simulink model "tests"  (R2013a)
settings: Solver=ode45  StartTime=0.0  StopTime=1  MaxStep=1e-3  RelTol=1e-3
undefined symbols (not defined in the file or in its folder): Nadc
libraries: simulink x1
settings Model: Creator=mainster  LastModifiedBy=mainster

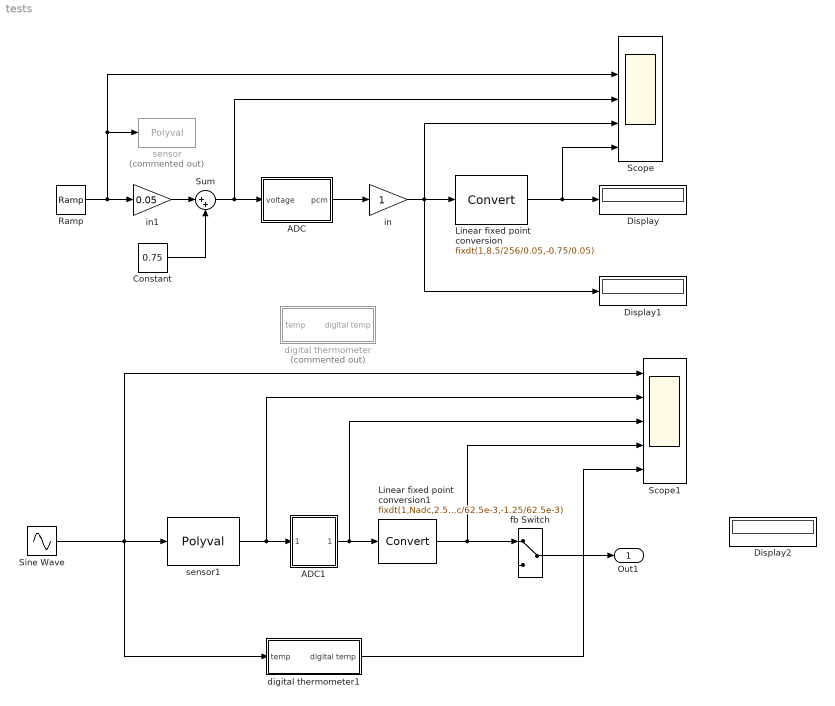
== system tests ==
  ADC : Subsystem
      mask Display: fprintf('ADC\n8-bit\n0-5V');
  ADC1 : Subsystem  mask{bypass=off}
      mask prompts: bypass "bypass adc"
      mask Callback bypass: %Simulink.Block.eval([gcb '/switch']);
      mask Display:
      | %fprintf('ADC\nGain=%s\n=%i',...
      | %    get_param([gcb '/scale'], 'Gain'),...
      | %    eval( get_param([gcb '/scale'], 'Gain') ));
      | if bypass
      |     color('red')
      |     fprintf('bypass\nADC')
      | else
      |     color('black')
      |     fprintf('ADC')
      | end
  Constant : Constant  Value=0.75
  Display : Display
  Display1 : Display
  Display2 : Display
  Linear fixed point conversion : DataTypeConversion  OutDataTypeStr=fixdt(1,8,5/256/0.05,-0.75/0.05)  ConvertRealWorld=Stored Integer (SI)
  Linear fixed point conversion1 : DataTypeConversion  OutDataTypeStr=fixdt(1,Nadc,2.5/2^Nadc/62.5e-3,-1.25/62.5e-3)  ConvertRealWorld=Stored Integer (SI)
  Ramp : simulink/Sources/Ramp  slope=50  start=0  X0=-5
  Scope : Scope  NumInputPorts=5
      settings: ShowLegends=on  TimeRange=1  YMin=-1~-10~0.5~0~-80  YMax=1~50~3~200~40
  Scope1 : Scope  NumInputPorts=5
      settings: ShowLegends=on  TimeRange=0.08057851239669417  YMin=-20~-10~-150~-3~-20  YMax=20~10~150~3~30
  Sine Wave : Sin  Amplitude=15  Frequency=2*pi  SampleTime=0
  Sum : Sum  Inputs=|++
  digital thermometer : Subsystem  Commented=on
  digital thermometer1 : Subsystem
  fb Switch : ManualSwitch
  in : Gain
  in1 : Gain  Gain=0.05
  sensor : Polyval  Commented=on  Coefs="[ 0.05     0.75 ]"
  sensor1 : Polyval  Coefs="[ 1/16    1.25]"
  Out1 : Outport
  wires:
  Linear fixed point conversion/1 -> Scope/5, Display/1
  ADC/1(pcm) -> in/1
  in/1 -> Scope/4, Display1/1, Linear fixed point conversion/1
  Ramp/1 -> Scope/2, sensor/1, in1/1
  Constant/1 -> Sum/2
  Sum/1 -> Scope/3, ADC/1(voltage)
  in1/1 -> Sum/1
  sensor1/1 -> ADC1/1(voltage), Scope1/2
  Sine Wave/1 -> digital thermometer1/1(temp), Scope1/1, sensor1/1
  fb Switch/1 -> Out1/1
  Linear fixed point conversion1/1 -> Scope1/4, fb Switch/1
  ADC1/1(pcm) -> Scope1/3, Linear fixed point conversion1/1
  digital thermometer1/1(digital temp) -> Scope1/5

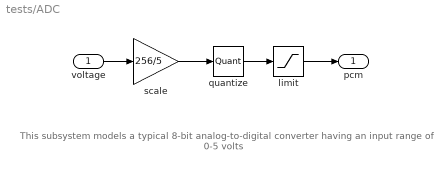
== system tests/ADC ==
  note: This subsystem models a typical
      | 8-bit analog-to-digital converter
      | having an input range of 0-5 volts
  voltage : Inport
  limit : Saturate  UpperLimit=255  LowerLimit=0
  quantize : Quantizer  QuantizationInterval=1
  scale : Gain  Gain=256/5  SaturateOnIntegerOverflow=on  OutDataTypeStr=Inherit: Same as input  ParamDataTypeStr=Inherit: Same as input
  pcm : Outport
  wires:
  limit/1 -> pcm/1
  scale/1 -> quantize/1
  quantize/1 -> limit/1
  voltage/1 -> scale/1

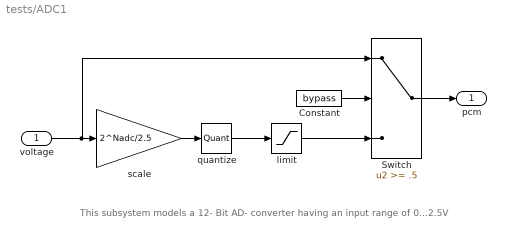
== system tests/ADC1 ==
  note: This subsystem models a 12- Bit AD- converter
      | having an input  range of 0...2.5V
  voltage : Inport
  Constant : Constant  Value=bypass
  Switch : Switch  Threshold=.5
  limit : Saturate  UpperLimit=2^Nadc-1  LowerLimit=0
  quantize : Quantizer
  scale : Gain  Gain=2^Nadc/2.5  SaturateOnIntegerOverflow=on  OutDataTypeStr=Inherit: Same as input  ParamDataTypeStr=Inherit: Same as input
  pcm : Outport
  wires:
  limit/1 -> Switch/3
  scale/1 -> quantize/1
  quantize/1 -> limit/1
  voltage/1 -> Switch/1, scale/1
  Constant/1 -> Switch/2
  Switch/1 -> pcm/1

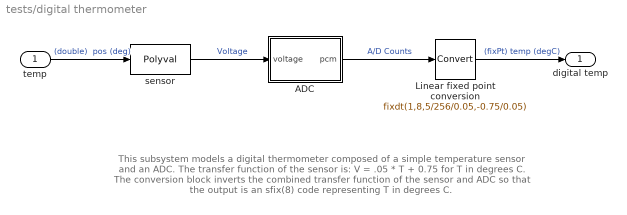
== system tests/digital thermometer ==
  note: This subsystem models a digital thermometer composed of a simple
      | temperature sensor and an ADC.  The transfer function of the sensor is:
      | V = .05 * T + 0.75
      | for T in degrees C.
      |
      | The conversion block inverts the combined transfer function of the sensor
      | and ADC so that the output is an sfix(8) code representing T in degrees C.
  temp : Inport
  ADC : Subsystem
      mask Display: fprintf('ADC\n8-bit\n0-5V');
  Linear fixed point conversion : DataTypeConversion  OutDataTypeStr=fixdt(1,8,5/256/0.05,-0.75/0.05)  ConvertRealWorld=Stored Integer (SI)
  sensor : Polyval  Coefs="[ 2     0 ]"
  digital temp : Outport
  wires:
  sensor/1 -> ADC/1(voltage)  "Voltage"
  ADC/1(pcm) -> Linear fixed point conversion/1  "A/D Counts"
  temp/1 -> sensor/1  "(double)  pos (deg)"
  Linear fixed point conversion/1 -> digital temp/1  "(fixPt) temp (degC)"

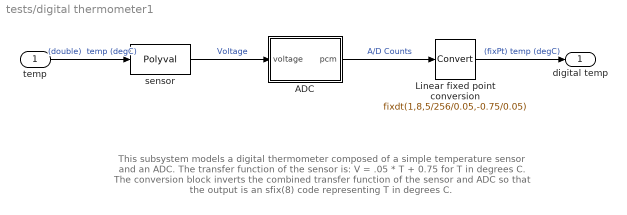
== system tests/digital thermometer1 ==
  note: This subsystem models a digital thermometer composed of a simple
      | temperature sensor and an ADC.  The transfer function of the sensor is:
      | V = .05 * T + 0.75
      | for T in degrees C.
      |
      | The conversion block inverts the combined transfer function of the sensor
      | and ADC so that the output is an sfix(8) code representing T in degrees C.
  temp : Inport
  ADC : Subsystem
      mask Display: fprintf('ADC\n8-bit\n0-5V');
  Linear fixed point conversion : DataTypeConversion  OutDataTypeStr=fixdt(1,8,5/256/0.05,-0.75/0.05)  ConvertRealWorld=Stored Integer (SI)
  sensor : Polyval  Coefs="[ 0.05     0.75 ]"
  digital temp : Outport
  wires:
  sensor/1 -> ADC/1(voltage)  "Voltage"
  ADC/1(pcm) -> Linear fixed point conversion/1  "A/D Counts"
  temp/1 -> sensor/1  "(double)  temp (degC)"
  Linear fixed point conversion/1 -> digital temp/1  "(fixPt) temp (degC)"

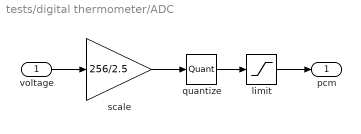
== system tests/digital thermometer/ADC ==
  voltage : Inport
  limit : Saturate  UpperLimit=255  LowerLimit=0
  quantize : Quantizer  QuantizationInterval=1
  scale : Gain  Gain=256/2.5  SaturateOnIntegerOverflow=on  OutDataTypeStr=Inherit: Same as input  ParamDataTypeStr=Inherit: Same as input
  pcm : Outport
  wires:
  limit/1 -> pcm/1
  scale/1 -> quantize/1
  quantize/1 -> limit/1
  voltage/1 -> scale/1

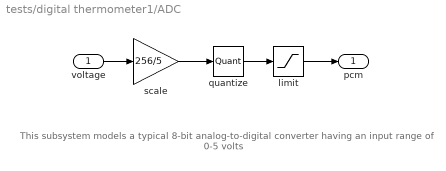
== system tests/digital thermometer1/ADC ==
  note: This subsystem models a typical
      | 8-bit analog-to-digital converter
      | having an input range of 0-5 volts
  voltage : Inport
  limit : Saturate  UpperLimit=255  LowerLimit=0
  quantize : Quantizer  QuantizationInterval=1
  scale : Gain  Gain=256/5  SaturateOnIntegerOverflow=on  OutDataTypeStr=Inherit: Same as input  ParamDataTypeStr=Inherit: Same as input
  pcm : Outport
  wires:
  limit/1 -> pcm/1
  scale/1 -> quantize/1
  quantize/1 -> limit/1
  voltage/1 -> scale/1
